simulink model "nonlinear_plant"  (R2019b)
settings: Solver=VariableStepAuto  StartTime=0.0  StopTime=800  FixedStep=1e-4  RelTol=1e-3
settings Model: Creator=Dhruv Laad  LastModifiedBy=Dhruv Laad

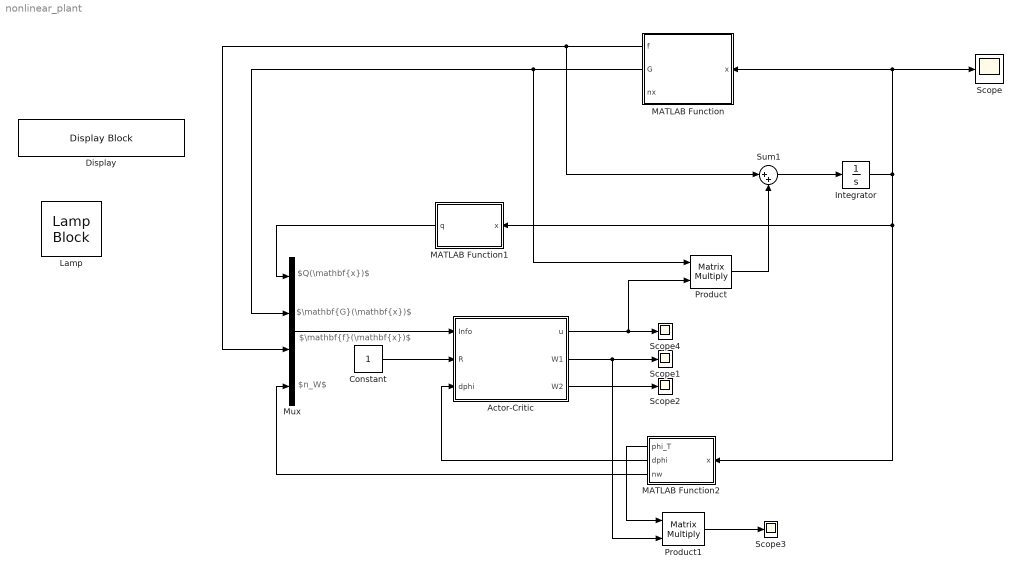
== system nonlinear_plant ==
  note: $n_W$
  note: $Q(\mathbf{x})$
  note: $\mathbf{G}(\mathbf{x})$
  note: $\mathbf{f}(\mathbf{x})$
  Actor-Critic : Subsystem
  Constant : Constant
  Display : DisplayBlock  LabelPosition=Hide  Format=short  Transparency=1
  Integrator : Integrator  InitialCondition=ones(3,1)
  Lamp : LampBlock  LabelPosition=Hide
  MATLAB Function : MATLAB Function  TreatAsAtomicUnit=on
  MATLAB Function1 : MATLAB Function  TreatAsAtomicUnit=on
  MATLAB Function2 : MATLAB Function  TreatAsAtomicUnit=on
  Mux : Mux
  Product : Product  Multiplication=Matrix(*)
  Product1 : Product  Multiplication=Matrix(*)
  Scope{,1..4} (5 alike) : Scope
  Sum1 : Sum  Inputs=|++
  wires:
  MATLAB Function1/1(q) -> Mux/1
  MATLAB Function/2(G) -> Product/1, Mux/2
  MATLAB Function/1(f) -> Sum1/1, Mux/3
  Actor-Critic/1(u) -> Scope4/1, Product/2
  Product/1 -> Sum1/2
  Sum1/1 -> Integrator/1
  Integrator/1 -> Scope/1, MATLAB Function/1(x), MATLAB Function2/1(x), MATLAB Function1/1(x)
  MATLAB Function2/3(nw) -> Mux/4
  Constant/1 -> Actor-Critic/2(R)
  Mux/1 -> Actor-Critic/1(Info)
  MATLAB Function2/2(dphi) -> Actor-Critic/3(dphi)
  Actor-Critic/2(W1) -> Product1/2, Scope1/1
  Actor-Critic/3(W2) -> Scope2/1
  MATLAB Function2/1(phi_T) -> Product1/1
  Product1/1 -> Scope3/1

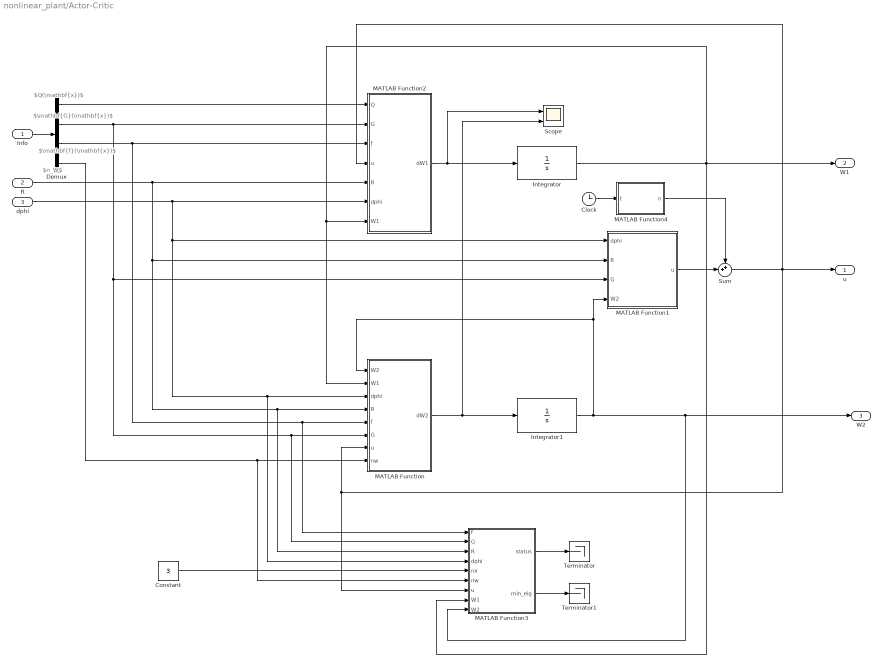
== system nonlinear_plant/Actor-Critic ==
  note: $\mathbf{f}(\mathbf{x})$
  note: $Q(\mathbf{x})$
  note: $n_W$
  note: $\mathbf{G}(\mathbf{x})$
  Info : Inport
  R : Inport  Port=2
  dphi : Inport  Port=3
  Clock : Clock
  Constant : Constant  Value=3
  Demux : Demux
  Integrator : Integrator  InitialCondition=ones(6,1)
  Integrator1 : Integrator  InitialCondition=ones(6,1)
  MATLAB Function : MATLAB Function  TreatAsAtomicUnit=on
  MATLAB Function1 : MATLAB Function  TreatAsAtomicUnit=on
  MATLAB Function2 : MATLAB Function  TreatAsAtomicUnit=on
  MATLAB Function3 : MATLAB Function  TreatAsAtomicUnit=on
  MATLAB Function4 : MATLAB Function  TreatAsAtomicUnit=on
  Scope : Scope  NumInputPorts=2
  Sum : Sum  Inputs=++|
  Terminator : Terminator
  Terminator1 : Terminator
  u : Outport
  W1 : Outport  Port=2
  W2 : Outport  Port=3
  wires:
  MATLAB Function/1(dW2) -> Scope/2, Integrator1/1
  Info/1 -> Demux/1
  Demux/1 -> MATLAB Function2/1(Q)
  Demux/2 -> MATLAB Function/6(G), MATLAB Function3/2(G), MATLAB Function1/3(G), MATLAB Function2/2(G)
  R/1 -> MATLAB Function3/3(R), MATLAB Function/4(R), MATLAB Function1/2(R), MATLAB Function2/5(R)
  dphi/1 -> MATLAB Function/3(dphi), MATLAB Function3/4(dphi), MATLAB Function1/1(dphi), MATLAB Function2/6(dphi)
  Demux/3 -> MATLAB Function/5(f), MATLAB Function3/1(f), MATLAB Function2/3(f)
  Demux/4 -> MATLAB Function3/6(nw), MATLAB Function/8(nw)
  MATLAB Function2/1(dW1) -> Scope/1, Integrator/1
  Integrator1/1 -> MATLAB Function3/9(W2), W2/1, MATLAB Function1/4(W2), MATLAB Function/1(W2)
  Integrator/1 -> MATLAB Function3/8(W1), MATLAB Function2/7(W1), MATLAB Function/2(W1), W1/1
  Constant/1 -> MATLAB Function3/5(nx)
  MATLAB Function3/1(status) -> Terminator/1
  MATLAB Function3/2(min_eig) -> Terminator1/1
  Clock/1 -> MATLAB Function4/1(t)
  MATLAB Function1/1(u) -> Sum/2
  MATLAB Function4/1(n) -> Sum/1
  Sum/1 -> MATLAB Function/7(u), MATLAB Function3/7(u), MATLAB Function2/4(u), u/1

== matlab function nonlinear_plant/MATLAB Function1 ==
  data: x input; q output
function q = Q(x)
    q = 10*x'*x;

== matlab function nonlinear_plant/MATLAB Function ==
  data: x input; f output; G output; nx output
function [f, G, nx] = dynamics(x)
    nx = 3;
    
%     x1 = x(1,1); x2 = x(2,1);
    
%     f = [-x1 + x2;
%          -0.5*x1 - 0.5*x2*(1 - (cos(2*x1) + 2)^2)];
%     
%     G = [0; cos(2*x1) + 2];
    A = [-1.01887,  0.90506, -0.00215;
      0.82225, -1.07741, -0.17555;
      0      ,  0      , -1];
    f = A*x;
    
    G = [0;0;1];

== matlab function nonlinear_plant/Actor-Critic/MATLAB Function2 ==
  data: Q input; G input size=[3 1]; f input size=[3 1]; u input size=1; dW1 output; R input; dphi input; W1 input
function dW1 = Critic(Q, G, f, u, R, dphi, W1)
    critic_lr = 1;

    sig_2 = dphi*(f + G*u);
    dW1 = -critic_lr*(sig_2/(sig_2'*sig_2 + 1)^2)*(sig_2'*W1 + Q + u'*R*u);

== matlab function nonlinear_plant/Actor-Critic/MATLAB Function ==
  data: W2 input; W1 input; dphi input; R input; f input; G input; u input; dW2 output; nw input
function dW2 = Actor(W2, W1, dphi, R, f, G, u, nw)
    actor_lr = 0.1;
    F2 = 4*eye(nw);
    F1 = 0.1*ones(nw,1);
    
    sig_2 = dphi*(f + G*u);
    D1 = dphi*G*(inv(R))*(G')*dphi';
    m = sig_2/(sig_2'*sig_2 + 1)^2;
    sig2_bar = sig_2/(sig_2'*sig_2 + 1);
    dW2 = -actor_lr *((F2*W2 - F1*sig2_bar'*W1) - 0.25*D1*W2*m'*W1);

== matlab function nonlinear_plant/Actor-Critic/MATLAB Function1 ==
  data: dphi input; R input; u output; G input; W2 input
function u = control_policy(dphi, R, G, W2)
    u = -0.5*(inv(R))*((G)')*(dphi')*W2;

== matlab function nonlinear_plant/MATLAB Function2 ==
  data: x input; phi_T output; dphi output; nw output
function [phi_T, dphi, nw] = basis(x)
    nw = 6;

    x1 = x(1,1); x2 = x(2,1); x3 = x(3);
    
%     phi = [x1^2; x1*x2; x2^2];
%     dphi = [2*x1, 0; x2, x1; 0, 2*x2];
    phi_T = [x1^2; x1*x2; x2^2; x2*x3; x3^2; x3*x1]';
    dphi = [2*x1,    0,    0; 
              x2,   x1,    0; 
               0, 2*x2,    0; 
               0,   x3,   x2;
               0,    0, 2*x3;
              x3,    0,   x1];

== matlab function nonlinear_plant/Actor-Critic/MATLAB Function3 ==
  data: f input; G input; R input; dphi input; nx input; nw input; u input; status output size=1; min_eig output size=1; W1 input; W2 input
function [status, min_eig] = check(f, G, R, dphi, nx, nw, u, W1, W2)
    q = 0.5;
    F2 = 1*eye(nw);
    F1 = 0*ones(nw,1);
    
    sig_2 = dphi*(f + G*u);
    D1 = dphi*G*(inv(R))*(G)'*dphi';
    ms = 1 + sig_2'*sig_2;
    m = sig_2/(sig_2'*sig_2 + 1)^2;

    M = [q*eye(nx), zeros(nx,1), zeros(nx, nw);
         zeros(1,nx), 1, (-0.5*F1 - (1/(8*ms))*D1*W1)';
         zeros(nw, nx), (-0.5*F1 - (1/(8*ms))*D1*W1), F2 - (1/8)*(D1*W1*m' + m*W2'*D1)];

    v = eig(M);
    min_eig = real(min(v));
    if min_eig <= 0
        status = 0;
    else
        status = 1;
    end
end

== matlab function nonlinear_plant/Actor-Critic/MATLAB Function4 ==
  data: t input; n output
function n = noise(t)
    if t <= 700
        n = 37*exp(-0.009*t)*(sin(t)^2*cos(t)+sin(2*t)^2*cos(0.1*t)+sin(-1.2*t)^2*cos(0.5*t)+sin(t)^5+sin(1.12*t)^2+cos(2.4*t)*sin(2.4*t)^3);
    else
        n = 0;
    end
